simulink model "simulinkmpc"  (R2018a)
settings: Solver=VariableStepAuto  StartTime=0.0  StopTime=50  RelTol=1e-3
settings Model: Creator=cemak  LastModifiedBy=cemak

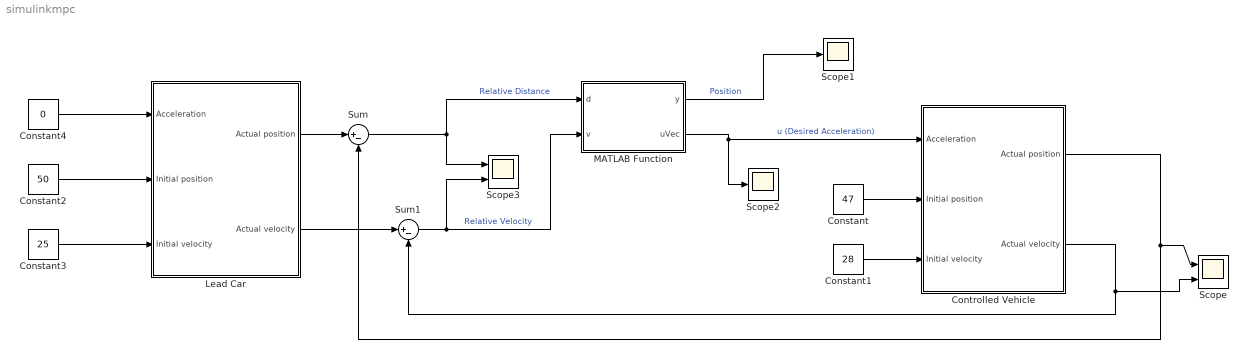
== system simulinkmpc ==
  Constant : Constant  Value=47
  Constant1 : Constant  Value=28
  Constant2 : Constant  Value=50
  Constant3 : Constant  Value=25
  Constant4 : Constant  Value=0
  Controlled Vehicle : Subsystem
  Lead Car : Subsystem
  MATLAB Function : MATLAB Function  TreatAsAtomicUnit=on
  Scope : Scope  NumInputPorts=2
  Scope1 : Scope
  Scope2 : Scope
  Scope3 : Scope  NumInputPorts=2
  Sum : Sum  Inputs=|+-
  Sum1 : Sum  Inputs=|+-
  wires:
  Constant/1 -> Controlled Vehicle/2(Initial position)
  Constant1/1 -> Controlled Vehicle/3(Initial velocity)
  Constant2/1 -> Lead Car/2(Initial position)
  Constant3/1 -> Lead Car/3(Initial velocity)
  Controlled Vehicle/1(Actual position) -> Scope/1, Sum/2
  Lead Car/2(Actual velocity) -> Sum1/1
  Controlled Vehicle/2(Actual velocity) -> Scope/2, Sum1/2
  Sum/1 -> Scope3/1, MATLAB Function/1(d)  "Relative Distance"
  Sum1/1 -> MATLAB Function/2(v), Scope3/2  "Relative Velocity"
  Constant4/1 -> Lead Car/1(Acceleration)
  MATLAB Function/2(uVec) -> Scope2/1, Controlled Vehicle/1(Acceleration)  "u (Desired Acceleration)"
  MATLAB Function/1(y) -> Scope1/1  "Position"
  Lead Car/1(Actual position) -> Sum/1

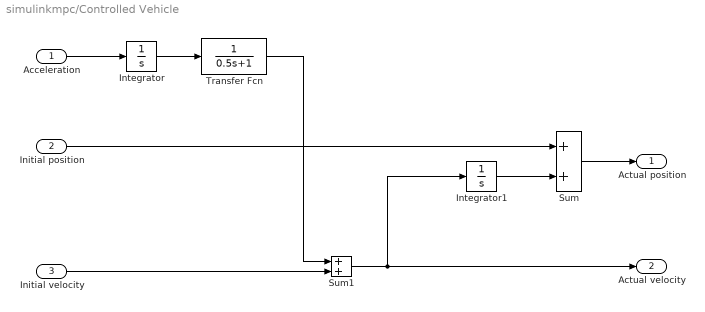
== system simulinkmpc/Controlled Vehicle ==
  Acceleration : Inport
  Initial position : Inport  Port=2
  Initial velocity : Inport  Port=3
  Integrator : Integrator
  Integrator1 : Integrator
  Sum : Sum
  Sum1 : Sum
  Transfer Fcn : TransferFcn  Denominator=[0.5 1]
  Actual position : Outport
  Actual velocity : Outport  Port=2
  wires:
  Sum1/1 -> Integrator1/1, Actual velocity/1
  Initial velocity/1 -> Sum1/2
  Sum/1 -> Actual position/1
  Transfer Fcn/1 -> Sum1/1
  Integrator/1 -> Transfer Fcn/1
  Acceleration/1 -> Integrator/1
  Initial position/1 -> Sum/1
  Integrator1/1 -> Sum/2

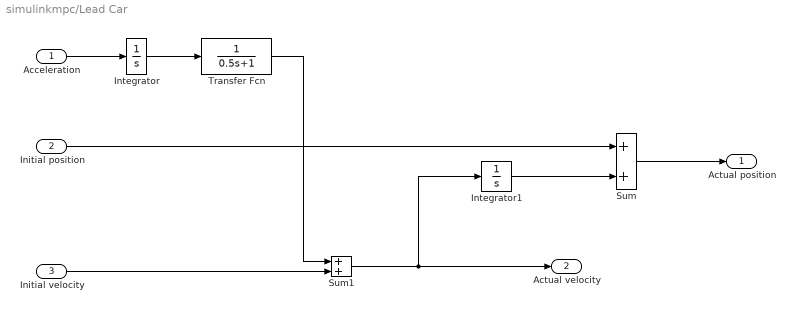
== system simulinkmpc/Lead Car ==
  Acceleration : Inport
  Initial position : Inport  Port=2
  Initial velocity : Inport  Port=3
  Integrator : Integrator
  Integrator1 : Integrator
  Sum : Sum
  Sum1 : Sum
  Transfer Fcn : TransferFcn  Denominator=[0.5 1]
  Actual position : Outport
  Actual velocity : Outport  Port=2
  wires:
  Transfer Fcn/1 -> Sum1/1
  Initial velocity/1 -> Sum1/2
  Sum/1 -> Actual position/1
  Integrator/1 -> Transfer Fcn/1
  Sum1/1 -> Integrator1/1, Actual velocity/1
  Acceleration/1 -> Integrator/1
  Initial position/1 -> Sum/1
  Integrator1/1 -> Sum/2

== matlab function simulinkmpc/MATLAB Function ==
  data: d input; y output; v input; uVec output
function [y,uVec] = fcn(d,v)
coder.extrinsic('quadprog');

xVec=zeros(3,1);
yVec=zeros();
Usol=zeros(4,1);
uVec = zeros(1,1);

A = [2.6 -2.21 0.6065; 1 0 0; 0 1 0];
B = [1; 0; 0];
C = [0.0023 0.0016 0.0001];
D = 0;
x0 = [d;v;0];
Ts = 0.1;
% Optimal control solution for $N = 4$
I = eye(3);
a=A*B;
b=A*A*B;
c=A*A*A*B;
G1 = [0 0 0 0 ; 0 0 0 0 ; 0 0 0 0];
G2 = [B(1) 0 0 0 ; B(2) 0 0 0 ; B(3) 0 0 0];
G3 = [a(1) B(1) 0 0 ; a(2) B(2) 0 0 ; a(3) B(3) 0 0];
G4 = [b(1) a(1) B(1) 0 ; b(2) a(2) B(2) 0;b(3) a(3) B(3) 0];
G5 = [c(1) b(1) a(1) B(1);c(2) b(2) a(2) B(2);c(3) b(3) a(3) B(3)];
G = [G1;G2;G3;G4;G5];
H = [I;A;A^2;A^3;A^4];
Q = C'*C;
R = 0.001;
% Q = eye(2);
Pinf = [0.0011 -0.0013 0.0004; -0.0013 0.0017 -0.0006; 0.0004 -0.0006 0.0002];
Kinf = inv(R+B'*Pinf*B)*B'*Pinf*A;
% A*X*A' - X + Q = 0; X = dlyap(A,Q)
P = Pinf;
Qf = P;
Qbar = blkdiag(Q,Q,Q,Q,Qf);
Rbar = blkdiag(R,R,R,R);
M = G'*Qbar*G + Rbar;
% input bound: umin <= u <= umax
umin = -5.5;
umax = 3;
lb = [umin;umin;umin;umin];
ub = [umax;umax;umax;umax];
% % Apply MPC steps
 xVec(:,1) = x0;
 %yVec(1) = C*x0;
 

 alpha = G'*Qbar*H*x0;
 Usol = quadprog(M,alpha',[],[],[],[],lb,ub);
 uVec(1) = Usol(1);
 xVec2 = A*xVec + b*uVec;
 yVec = C*xVec;
%  
%       alpha = G'*Qbar*H*xVec(:,k);
    %   Usol(1) = quadprog(M,alpha',[],[],[],[],lb,ub);
      % uVec(1) = Usol(1);
%       xVec(1) = A*xVec(1) + B*uVec(1);
%       yVec(1) = C*xVec(1);
 %X2 = A*x0+ B*Usol;

% u=Usol(1);

y = yVec;
